simulink library "T_Sensor"  (R2018b)
settings: Solver=ode45  StartTime=0.0  StopTime=10.0  RelTol=1e-3  EnableMultiTasking=on
settings Model: Creator=lena.frank  LastModifiedBy=P41573
settings DataIOCC: LimitDataPoints=on  SaveFormat=Array  SignalLoggingSaveFormat=ModelDataLogs
settings OptimizationCC: ExpressionDepthLimit=2147483647  LifeSpan=inf
settings DebuggingCC: UnderspecifiedInitializationDetection=Classic  MergeDetectMultiDrivingBlocksExec=none  SolverPrmCheckMsg=warning  FcnCallInpInsideContextMsg=warning  StateNameClashWarn=warning  SFUnexpectedBacktrackingDiag=warning  SFNoUnconditionalDefaultTransitionDiag=warning  SFExecutionAtInitializationDiag=none
settings HardwareCC: ProdBitPerPointer=32  ProdBitPerSizeT=32  ProdBitPerPtrDiffT=32  ProdLargestAtomicFloat=None  ProdIntDivRoundTo=Undefined  ProdEndianess=Unspecified  ProdWordSize=32  ProdHWDeviceType=32-bit Generic
settings ModelReferenceCC: PropagateSignalLabelsOutOfModel=off
settings SFSimCC: SimUseLocalCustomCode=off
settings RTWCC: RTWUseLocalCustomCode=off
settings CodeAppCC: StateflowObjectComments=on
settings GRTTargetCC: TargetLangStandard=C89/C90 (ANSI)  GeneratePreprocessorConditionals=Disable all  CombineOutputUpdateFcns=off  GRTInterface=on
settings ConfigComp: CovMetricSettings=dw  CovHtmlReporting=on  CovSaveCumulativeToWorkspaceVar=on  CovSaveSingleToWorkspaceVar=on  CovExternalEMLEnable=off

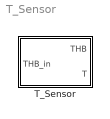
== system T_Sensor ==
  T_Sensor : Subsystem  mask(temperature measurement sensor){tc=10, t0=20}
      mask prompts: tc "time constant of sensor [s]"; t0 "initial temperature [degree centigrade]"
      mask help: Measurement sensor for temperatures with first-oder hold. Temperature is in degree centigrade.
      mask init:
      | tc = 1/max(tc, 0.001);
      mask Help: web(fullfile(path_carnot('help'),'T_Sensor.html'),'-helpbrowser')
      mask Display: plot(0,0,100,100,[50,55,65,70,70,65,55,45,35,30,30,35,44,50,50],[50,50,60,70,80,90,100,100,90,80,70,60,50,50,-0],[60,40],[90,90],[50,50],[57,90])

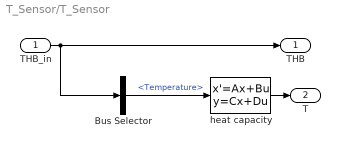
== system T_Sensor/T_Sensor ==
  THB_in : Inport
  Bus Selector : BusSelector  OutputSignals=Temperature
  heat capacity : StateSpace  A=-tc  B=tc  D=0  InitialCondition=t0
  THB : Outport
  T : Outport  Port=2
  wires:
  heat capacity/1 -> T/1
  Bus Selector/1 -> heat capacity/1  "<Temperature>"
  THB_in/1 -> Bus Selector/1, THB/1
